simulink model "CubeQuat"  (R2014a)
settings: Solver=ode45  StartTime=0.0  StopTime=10  RelTol=1e-3
values from neighbouring files (symbols this model uses):
  euler_init = [0;0;0]    [CubeQuat_setup.m]
  I = diag([10;10;10])    [CubeQuat_setup.m]
  k = 40    [CubeQuat_setup.m]
  kd = 2*sqrt(I(1,1))*sqrt(kp)    [CubeQuat_setup.m]
  kp = 40    [CubeQuat_setup.m]
  M = zeros(3,1)    [CubeQuat_setup.m]
  omega_0 = [0;0;0]    [CubeQuat_setup.m]
  x_0 = [0,0,0,1,0,0,0]    [CubeQuat_setup.m]
libraries: cstblocks x6, aerolibtransform2 x5, dspsigops x1
settings Model: Creator=Daire  LastModifiedBy=Daire

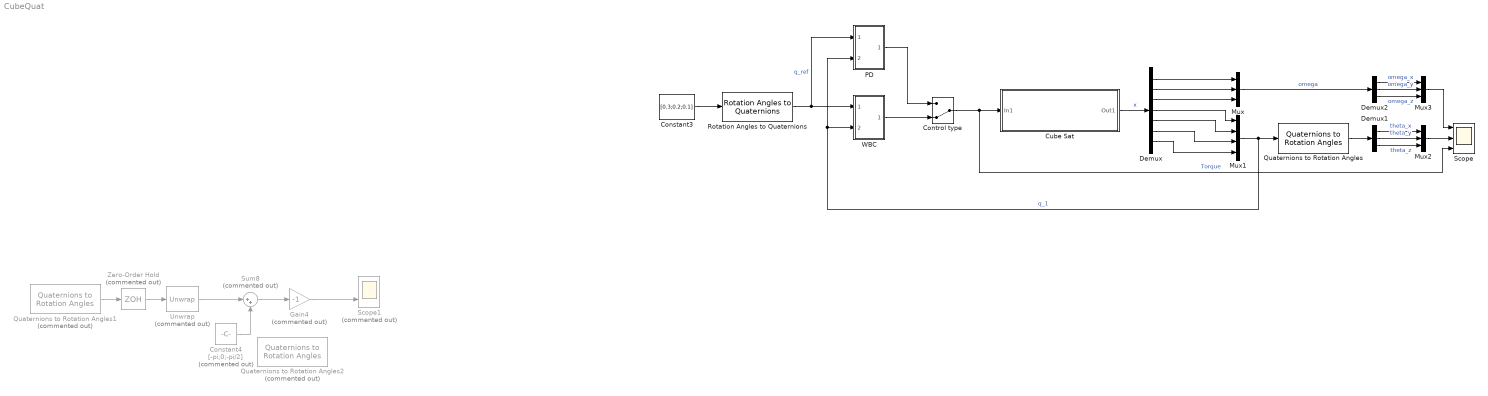
== system CubeQuat ==
  Constant3 : Constant  Value=[0.3;0.2;0.1]
  Constant4 : Constant  Commented=on  Value=[-pi;0;-pi/2]
  Control type : ManualSwitch  CurrentSetting=0
  Cube Sat : Subsystem
  Demux : Demux  Outputs=7
  Demux1 : Demux  Outputs=3
  Demux2 : Demux  Outputs=3
  Gain4 : Gain  Commented=on  Gain=-1
  Mux : Mux  Inputs=3
  Mux1 : Mux
  Mux2 : Mux  Inputs=3
  Mux3 : Mux  Inputs=3
  PD : Subsystem
  Quaternions to Rotation Angles : aerolibtransform2/Quaternions to Rotation Angles  rotationOrder=ZYX
  Quaternions to Rotation Angles1 : aerolibtransform2/Quaternions to Rotation Angles  Commented=on  rotationOrder=ZYX
  Quaternions to Rotation Angles2 : aerolibtransform2/Quaternions to Rotation Angles  Commented=on  rotationOrder=ZYX
  Rotation Angles to Quaternions : aerolibtransform2/Rotation Angles to Quaternions  rotationOrder=ZYX
  Scope : Scope  NumInputPorts=3
      settings: ShowLegends=on  YMin=-0.7~-0.275~-5  YMax=0.4~0~5
  Scope1 : Scope  Commented=on  NumInputPorts=2
      settings: ShowLegends=on  YMin=-3.5~-3.5  YMax=3.5~3.5
  Sum8 : Sum  Commented=on  Inputs=|++
  Unwrap : dspsigops/Unwrap  Commented=on  tol=pi  running=off
  WBC : Subsystem
  Zero-Order Hold : ZeroOrderHold  Commented=on  SampleTime=0.001
  wires:
  Demux/1 -> Mux/1
  Demux/2 -> Mux/2
  Demux/3 -> Mux/3
  Demux/4 -> Mux1/1
  Demux/5 -> Mux1/2
  Demux/6 -> Mux1/3
  Demux/7 -> Mux1/4
  Mux1/1 -> Quaternions to Rotation Angles/1, PD/2(In2), WBC/2(In2)  "q_1"
  Quaternions to Rotation Angles/1 -> Demux1/1
  Rotation Angles to Quaternions/1 -> PD/1(In1), WBC/1(In1)  "q_ref"
  Constant3/1 -> Rotation Angles to Quaternions/1
  Demux1/1 -> Mux2/1  "theta_x"
  Demux1/2 -> Mux2/2  "theta_y"
  Demux1/3 -> Mux2/3  "theta_z"
  Mux2/1 -> Scope/2
  Mux/1 -> Demux2/1  "omega"
  Demux2/1 -> Mux3/1  "omega_x"
  Demux2/2 -> Mux3/2  "omega_y"
  Demux2/3 -> Mux3/3  "omega_z"
  Mux3/1 -> Scope/1
  ? -> Quaternions to Rotation Angles1/1
  Quaternions to Rotation Angles1/1 -> Zero-Order Hold/1
  Sum8/1 -> Gain4/1
  Zero-Order Hold/1 -> Unwrap/1
  Constant4/1 -> Sum8/2
  Unwrap/1 -> Sum8/1
  Gain4/1 -> Scope1/2
  WBC/1(Out1) -> Control type/2
  Cube Sat/1(Out1) -> Demux/1  "x"
  Control type/1 -> Scope/3, Cube Sat/1(In1)  "Torque"
  PD/1(Out1) -> Control type/1

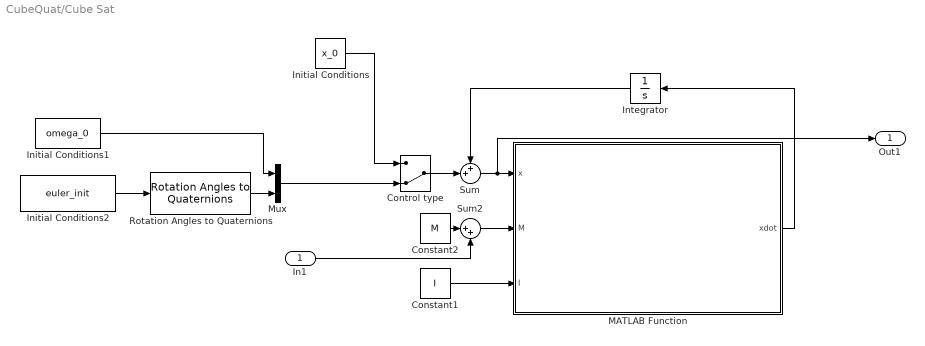
== system CubeQuat/Cube Sat ==
  In1 : Inport
  Constant1 : Constant  Value=I
  Constant2 : Constant  Value=M
  Control type : ManualSwitch  CurrentSetting=0
  Initial Conditions : Constant  Value=x_0
  Initial Conditions1 : Constant  Value=omega_0
  Initial Conditions2 : Constant  Value=euler_init
  Integrator : Integrator
  MATLAB Function : MATLAB Function  TreatAsAtomicUnit=on
  Mux : Mux  Inputs=2
  Rotation Angles to Quaternions : aerolibtransform2/Rotation Angles to Quaternions  rotationOrder=ZYX
  Sum : Sum  Inputs=++|
  Sum2 : Sum  Inputs=|++
  Out1 : Outport
  wires:
  Sum2/1 -> MATLAB Function/2(M)
  Sum/1 -> Out1/1, MATLAB Function/1(x)
  Integrator/1 -> Sum/1
  Constant2/1 -> Sum2/1
  Constant1/1 -> MATLAB Function/3(I)
  Control type/1 -> Sum/2
  MATLAB Function/1(xdot) -> Integrator/1
  In1/1 -> Sum2/2
  Rotation Angles to Quaternions/1 -> Mux/2
  Initial Conditions1/1 -> Mux/1
  Initial Conditions2/1 -> Rotation Angles to Quaternions/1
  Mux/1 -> Control type/2
  Initial Conditions/1 -> Control type/1

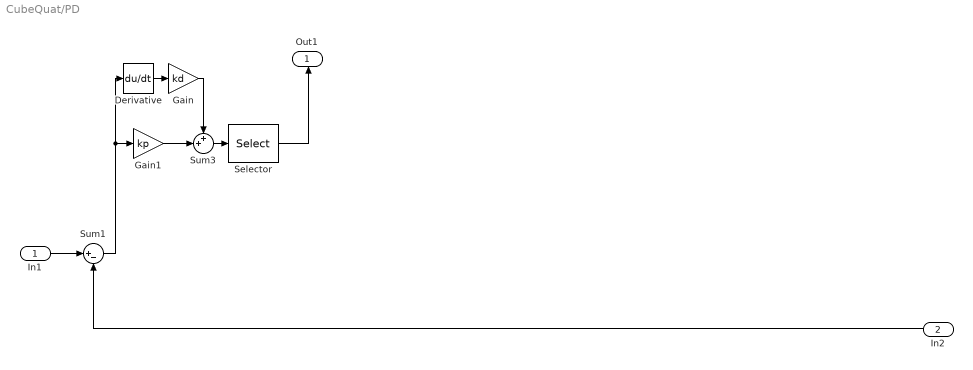
== system CubeQuat/PD ==
  In1 : Inport
  In2 : Inport  Port=2
  Derivative : Derivative
  Gain : Gain  Gain=kd
  Gain1 : Gain  Gain=kp
  Selector : Selector  InputPortWidth=4  Indices=[2,3,4]
  Sum1 : Sum  Inputs=|+-
  Sum3 : Sum  Inputs=++|
  Out1 : Outport
  wires:
  Selector/1 -> Out1/1
  Gain/1 -> Sum3/1
  Derivative/1 -> Gain/1
  Gain1/1 -> Sum3/2
  Sum1/1 -> Gain1/1, Derivative/1
  In2/1 -> Sum1/2
  In1/1 -> Sum1/1
  Sum3/1 -> Selector/1

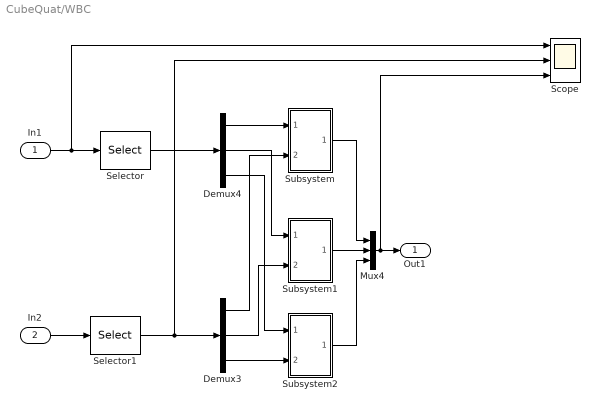
== system CubeQuat/WBC ==
  In1 : Inport
  In2 : Inport  Port=2
  Demux3 : Demux  Outputs=3
  Demux4 : Demux  Outputs=3
  Mux4 : Mux  Inputs=3
  Scope : Scope  NumInputPorts=3
      settings: ShowLegends=on  TimeRange=10  YMin=-0.7~-0.275~-5  YMax=0.4~0~5  SaveName=ScopeData2
  Selector : Selector  InputPortWidth=4  Indices=[2,3,4]
  Selector1 : Selector  InputPortWidth=4  Indices=[2,3,4]
  Subsystem : Subsystem
  Subsystem1 : Subsystem
  Subsystem2 : Subsystem
  Out1 : Outport
  wires:
  Demux3/3 -> Subsystem2/2(In2)
  In2/1 -> Selector1/1
  Demux4/1 -> Subsystem/1(In1)
  Demux4/3 -> Subsystem2/1(In1)
  Subsystem1/1(Out1) -> Mux4/2
  Mux4/1 -> Scope/3, Out1/1
  Subsystem2/1(Out1) -> Mux4/3
  Subsystem/1(Out1) -> Mux4/1
  In1/1 -> Selector/1, Scope/1
  Selector/1 -> Demux4/1
  Demux4/2 -> Subsystem1/1(In1)
  Selector1/1 -> Scope/2, Demux3/1
  Demux3/2 -> Subsystem1/2(In2)
  Demux3/1 -> Subsystem/2(In2)

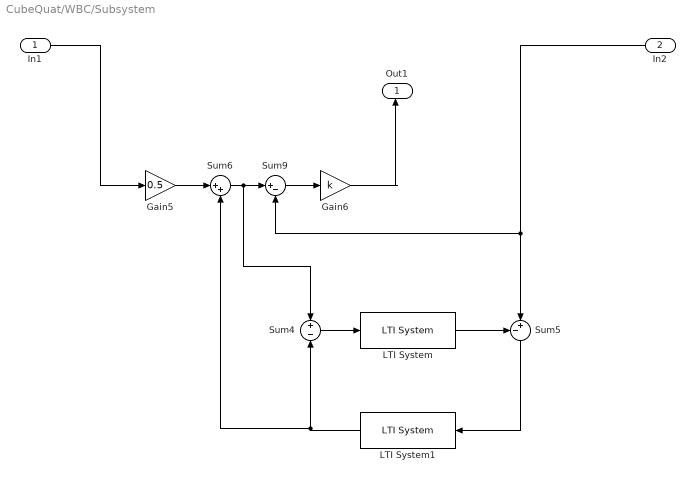
== system CubeQuat/WBC/Subsystem ==
  In1 : Inport
  In2 : Inport  Port=2
  Gain5 : Gain  Gain=0.5
  Gain6 : Gain  Gain=k
  LTI System : cstblocks/LTI System  sys=G  IC=[]
  LTI System1 : cstblocks/LTI System  sys=G  IC=[]
  Sum4 : Sum  Inputs=+|-
  Sum5 : Sum  Inputs=-+|
  Sum6 : Sum  Inputs=|++
  Sum9 : Sum  Inputs=|+-
  Out1 : Outport
  wires:
  Sum6/1 -> Sum4/1, Sum9/1
  In1/1 -> Gain5/1
  Sum9/1 -> Gain6/1
  Gain6/1 -> Out1/1
  Gain5/1 -> Sum6/1
  LTI System1/1 -> Sum6/2, Sum4/2
  Sum4/1 -> LTI System/1
  LTI System/1 -> Sum5/1
  Sum5/1 -> LTI System1/1
  In2/1 -> Sum9/2, Sum5/2

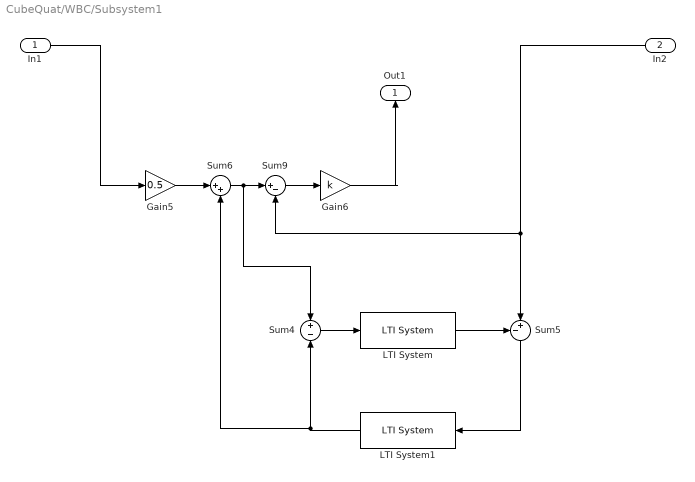
== system CubeQuat/WBC/Subsystem1 ==
  In1 : Inport
  In2 : Inport  Port=2
  Gain5 : Gain  Gain=0.5
  Gain6 : Gain  Gain=k
  LTI System : cstblocks/LTI System  sys=G  IC=[]
  LTI System1 : cstblocks/LTI System  sys=G  IC=[]
  Sum4 : Sum  Inputs=+|-
  Sum5 : Sum  Inputs=-+|
  Sum6 : Sum  Inputs=|++
  Sum9 : Sum  Inputs=|+-
  Out1 : Outport
  wires:
  In2/1 -> Sum5/2, Sum9/2
  Sum5/1 -> LTI System1/1
  LTI System/1 -> Sum5/1
  Sum4/1 -> LTI System/1
  LTI System1/1 -> Sum4/2, Sum6/2
  Gain5/1 -> Sum6/1
  Gain6/1 -> Out1/1
  Sum9/1 -> Gain6/1
  In1/1 -> Gain5/1
  Sum6/1 -> Sum9/1, Sum4/1

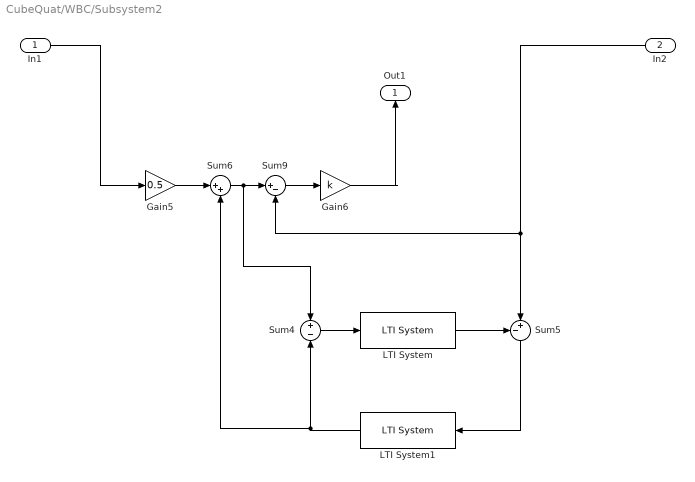
== system CubeQuat/WBC/Subsystem2 ==
  In1 : Inport
  In2 : Inport  Port=2
  Gain5 : Gain  Gain=0.5
  Gain6 : Gain  Gain=k
  LTI System : cstblocks/LTI System  sys=G  IC=[]
  LTI System1 : cstblocks/LTI System  sys=G  IC=[]
  Sum4 : Sum  Inputs=+|-
  Sum5 : Sum  Inputs=-+|
  Sum6 : Sum  Inputs=|++
  Sum9 : Sum  Inputs=|+-
  Out1 : Outport
  wires:
  Sum6/1 -> Sum4/1, Sum9/1
  In1/1 -> Gain5/1
  Sum9/1 -> Gain6/1
  Gain6/1 -> Out1/1
  Gain5/1 -> Sum6/1
  LTI System1/1 -> Sum6/2, Sum4/2
  Sum4/1 -> LTI System/1
  LTI System/1 -> Sum5/1
  Sum5/1 -> LTI System1/1
  In2/1 -> Sum9/2, Sum5/2

== matlab function CubeQuat/Cube Sat/MATLAB Function ==
  data: x input; xdot output; M input; I input
function xdot = CubeQuat(x,M,I)
%UNTITLED3 Summary of this function goes here
%   Detailed explanation goes here

%x=[e1,e2,e3,e1dot,e2dot,e3dot];

omega=x(1:3);
q=x(4:7);
n=q(1);
eta=q(2:4);

S=SkewSym(eta);
%R=quat2dcm(q);


omega_dot=I\((-cross(omega,I*omega))+M);
ndot=-0.5*transpose(eta)*omega;
etadot=0.5*((n*eye(3))+S)*omega;

xdot=[omega_dot;ndot;etadot];


end
